simulink model "Medium_Intro_Lab"  (R2022b)
settings: Solver=VariableStepAuto  StartTime=0.0  StopTime=10.0  MaxStep=1e-3  RelTol=1e-3
libraries: simulink x1
settings Model: Creator=LOQ  LastModifiedBy=LOQ
settings OptimizationCC: ReuseModelBlockBuffer=on
settings RTWCC: GPUComputeCapability=5.0
settings ConfigComp: CovBoundaryAbsTol=1.0e-5

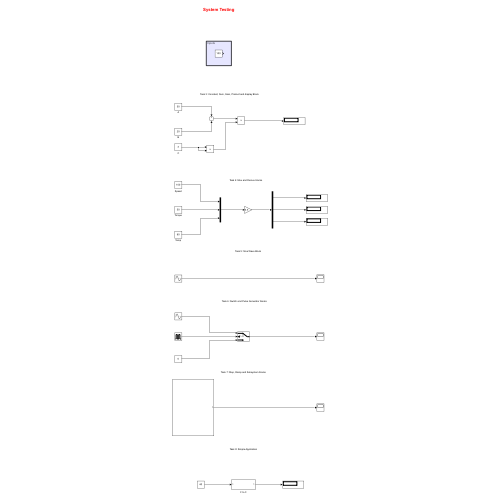
[thumbnail: Simulink's stored preview of the top-level diagram]
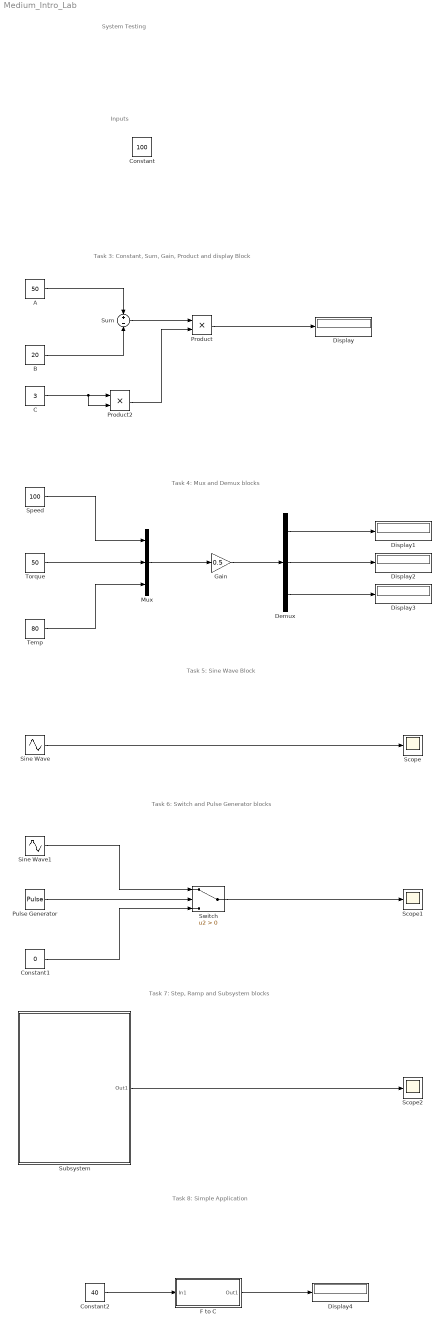
== system Medium_Intro_Lab ==
  note: Task 8: Simple Application
  note: Task 7: Step, Ramp and Subsystem blocks
  note: Task 6: Switch and Pulse Generator blocks
  note: Task 5: Sine Wave Block
  note: Task 4: Mux and Demux blocks
  note: Task 3: Constant, Sum, Gain, Product and display Block
  note: System Testing
  note: Inputs
  A : Constant  Value=50
  B : Constant  Value=20
  C : Constant  Value=3
  Constant : Constant  Value=100
  Constant1 : Constant  Value=0
  Constant2 : Constant  Value=40
  Demux : Demux  Outputs=3
  Display{,1..4} (5 alike) : Display
  F to C : Subsystem
  Gain : Gain  Gain=0.5
  Mux : Mux  Inputs=3
  Product : Product
  Product2 : Product
  Pulse Generator : DiscretePulseGenerator  PulseType=Time based  PulseWidth=50
  Scope : Scope
  Scope1 : Scope
  Scope2 : Scope
  Sine Wave : Sin  Amplitude=10  Frequency=5  Phase=pi/2  SampleTime=0
  Sine Wave1 : Sin  Amplitude=5  Frequency=10  SampleTime=0
  Speed : Constant  Value=100
  Subsystem : Subsystem
  Sum : Sum  Inputs=+-
  Switch : Switch  Criteria=u2 > Threshold  SaturateOnIntegerOverflow=off  InputSameDT=off
  Temp : Constant  Value=80
  Torque : Constant  Value=50
  wires:
  A/1 -> Sum/1
  B/1 -> Sum/2
  Sum/1 -> Product/1
  Product/1 -> Display/1
  C/1 -> Product2/2, Product2/1
  Product2/1 -> Product/2
  Torque/1 -> Mux/2
  Speed/1 -> Mux/1
  Temp/1 -> Mux/3
  Gain/1 -> Demux/1
  Mux/1 -> Gain/1
  Demux/1 -> Display1/1
  Demux/3 -> Display3/1
  Demux/2 -> Display2/1
  Sine Wave/1 -> Scope/1
  Sine Wave1/1 -> Switch/1
  Pulse Generator/1 -> Switch/2
  Constant1/1 -> Switch/3
  Switch/1 -> Scope1/1
  Subsystem/1(Out1) -> Scope2/1
  Constant2/1 -> F to C/1(In1)
  F to C/1(Out1) -> Display4/1

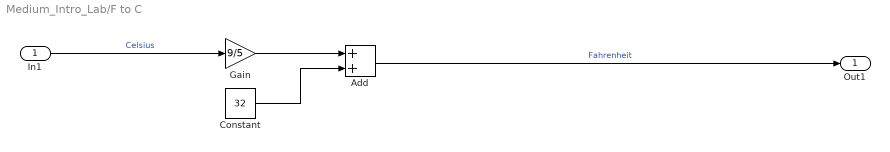
== system Medium_Intro_Lab/F to C ==
  In1 : Inport
  Add : Sum
  Constant : Constant  Value=32
  Gain : Gain  Gain=9/5
  Out1 : Outport
  wires:
  Gain/1 -> Add/1
  Constant/1 -> Add/2
  In1/1 -> Gain/1  "Celsius"
  Add/1 -> Out1/1  "Fahrenheit"

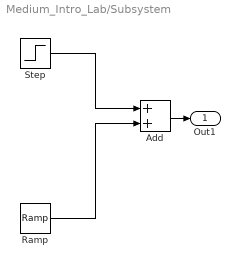
== system Medium_Intro_Lab/Subsystem ==
  Add : Sum
  Ramp : simulink/Sources/Ramp  slope=3  start=2  InitialOutput=0
  Step : Step  Time=2  After=5  SampleTime=0
  Out1 : Outport
  wires:
  Step/1 -> Add/1
  Add/1 -> Out1/1
  Ramp/1 -> Add/2
